simulink model "tema2_mdl_pin"  (R2019a)
settings: Solver=VariableStepAuto  StartTime=0.0  StopTime=400  RelTol=1e-3
settings Model: Creator=cynthia  LastModifiedBy=cynthia

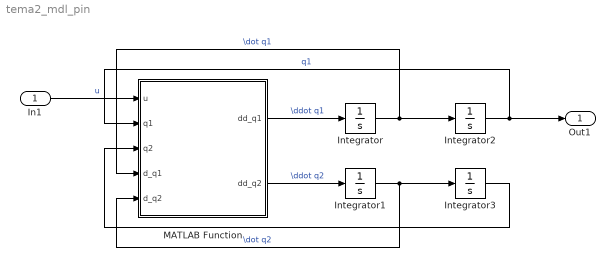
== system tema2_mdl_pin ==
  In1 : Inport
  Integrator{,1..3} (4 alike) : Integrator
  MATLAB Function : MATLAB Function  TreatAsAtomicUnit=on
  Out1 : Outport
  wires:
  MATLAB Function/1(dd_q1) -> Integrator/1  "\\ddot q1"
  Integrator/1 -> Integrator2/1, MATLAB Function/4(d_q1)  "\\dot q1"
  MATLAB Function/2(dd_q2) -> Integrator1/1  "\\ddot q2"
  Integrator1/1 -> Integrator3/1, MATLAB Function/5(d_q2)  "\\dot q2"
  In1/1 -> MATLAB Function/1(u)  "u"
  Integrator2/1 -> MATLAB Function/2(q1), Out1/1  "q1"
  Integrator3/1 -> MATLAB Function/3(q2)

== matlab function tema2_mdl_pin/MATLAB Function ==
  data: u input; dd_q1 output; q1 input; q2 input; d_q1 input; d_q2 input; dd_q2 output
function [dd_q1,dd_q2] = fcn(u,q1,q2,d_q1,d_q2)
m = 5.1;
g = 10;
L = 1.56;
zeta = 7.64;
k = 0.25;
J = 2.77; 
I = 1.89;
M = 2.82;

dd_q1 = (u + k*(q2-q1) - zeta*d_q1)/J;
dd_q2 = (-M*g*L*sin(q2) - k*(q2-q1) - zeta*d_q2)/I;


end
